simulink model "StabilityControlSystemMessy"  (R2023a)
settings: Solver=VariableStepAuto  StartTime=0.0  StopTime=10.0  RelTol=1e-3
libraries: simulink x2, slpidlib x1
settings Model: Creator=edill  LastModifiedBy=harshs
settings RTWCC: GPUComputeCapability=5.0
settings ConfigComp: CovBoundaryAbsTol=1.0e-5

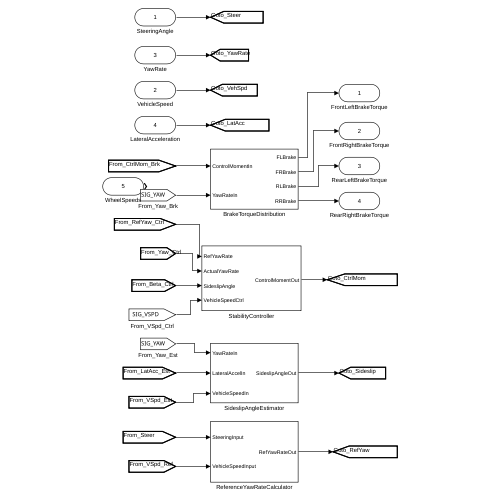
[thumbnail: Simulink's stored preview of the top-level diagram]
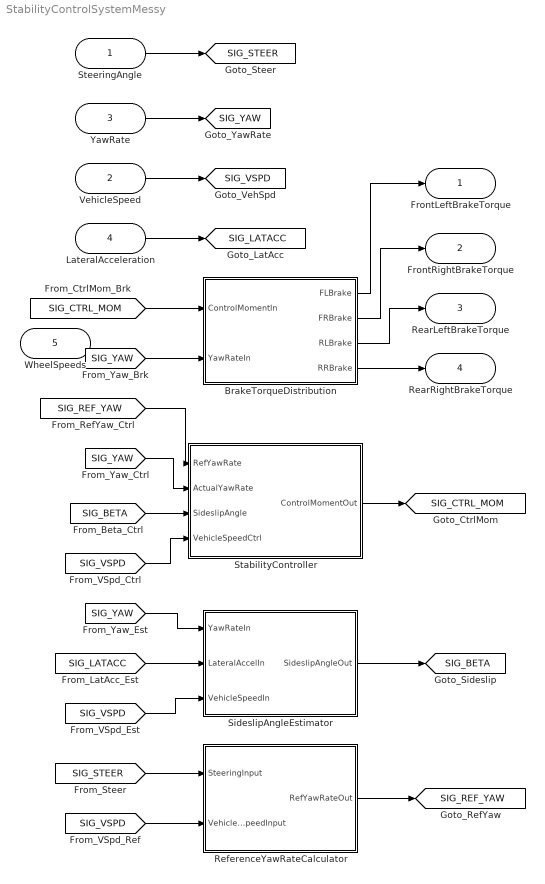
== system StabilityControlSystemMessy ==
  SteeringAngle : Inport
  VehicleSpeed : Inport  Port=2
  YawRate : Inport  Port=3
  LateralAcceleration : Inport  Port=4
  WheelSpeeds : Inport  Port=5  PortDimensions=4
  BrakeTorqueDistribution : Subsystem
  ReferenceYawRateCalculator : Subsystem
  SideslipAngleEstimator : Subsystem
  StabilityController : Subsystem
  FrontLeftBrakeTorque : Outport
  FrontRightBrakeTorque : Outport  Port=2
  RearLeftBrakeTorque : Outport  Port=3
  RearRightBrakeTorque : Outport  Port=4
  tag scope: SIG_BETA=global, SIG_CTRL_MOM=global, SIG_LATACC=global, SIG_REF_YAW=global, SIG_STEER=global, SIG_VSPD=global, SIG_YAW=global
  wires:
  [SIG_CTRL_MOM] -> BrakeTorqueDistribution/1(ControlMomentIn)
  VehicleSpeed/1 -> [SIG_VSPD]
  SteeringAngle/1 -> [SIG_STEER]
  ReferenceYawRateCalculator/1(RefYawRateOut) -> [SIG_REF_YAW]
  YawRate/1 -> [SIG_YAW]
  [SIG_YAW] -> StabilityController/2(ActualYawRate)
  LateralAcceleration/1 -> [SIG_LATACC]
  [SIG_YAW] -> BrakeTorqueDistribution/2(YawRateIn)
  [SIG_VSPD] -> SideslipAngleEstimator/3(VehicleSpeedIn)
  [SIG_REF_YAW] -> StabilityController/1(RefYawRate)
  [SIG_BETA] -> StabilityController/3(SideslipAngle)
  [SIG_VSPD] -> StabilityController/4(VehicleSpeedCtrl)
  [SIG_YAW] -> SideslipAngleEstimator/1(YawRateIn)
  [SIG_LATACC] -> SideslipAngleEstimator/2(LateralAccelIn)
  [SIG_STEER] -> ReferenceYawRateCalculator/1(SteeringInput)
  [SIG_VSPD] -> ReferenceYawRateCalculator/2(VehicleSpeedInput)
  BrakeTorqueDistribution/1(FLBrake) -> FrontLeftBrakeTorque/1
  BrakeTorqueDistribution/2(FRBrake) -> FrontRightBrakeTorque/1
  BrakeTorqueDistribution/3(RLBrake) -> RearLeftBrakeTorque/1
  BrakeTorqueDistribution/4(RRBrake) -> RearRightBrakeTorque/1
  StabilityController/1(ControlMomentOut) -> [SIG_CTRL_MOM]
  SideslipAngleEstimator/1(SideslipAngleOut) -> [SIG_BETA]

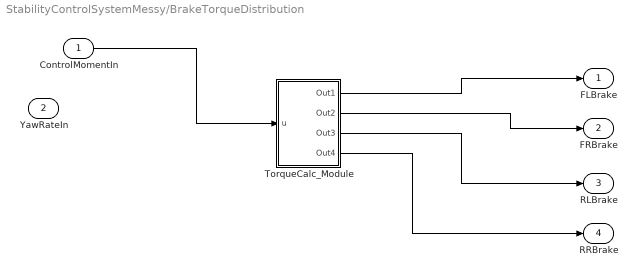
== system StabilityControlSystemMessy/BrakeTorqueDistribution ==
  ControlMomentIn : Inport
  YawRateIn : Inport  Port=2
  TorqueCalc_Module : Subsystem
  FLBrake : Outport
  FRBrake : Outport  Port=2
  RLBrake : Outport  Port=3
  RRBrake : Outport  Port=4
  wires:
  ControlMomentIn/1 -> TorqueCalc_Module/1(u)
  TorqueCalc_Module/1(Out1) -> FLBrake/1
  TorqueCalc_Module/2(Out2) -> FRBrake/1
  TorqueCalc_Module/3(Out3) -> RLBrake/1
  TorqueCalc_Module/4(Out4) -> RRBrake/1

== system StabilityControlSystemMessy/ReferenceYawRateCalculator ==
  SteeringInput : Inport
  VehicleSpeedInput : Inport  Port=2
  YawRateCalc_Core : Subsystem
  RefYawRateOut : Outport
  wires:
  SteeringInput/1 -> YawRateCalc_Core/1(In1)
  VehicleSpeedInput/1 -> YawRateCalc_Core/2(In2)
  YawRateCalc_Core/1(Out1) -> RefYawRateOut/1

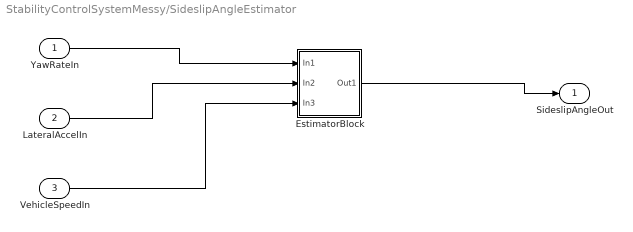
== system StabilityControlSystemMessy/SideslipAngleEstimator ==
  YawRateIn : Inport
  LateralAccelIn : Inport  Port=2
  VehicleSpeedIn : Inport  Port=3
  EstimatorBlock : Subsystem
  SideslipAngleOut : Outport
  wires:
  YawRateIn/1 -> EstimatorBlock/1(In1)
  LateralAccelIn/1 -> EstimatorBlock/2(In2)
  VehicleSpeedIn/1 -> EstimatorBlock/3(In3)
  EstimatorBlock/1(Out1) -> SideslipAngleOut/1

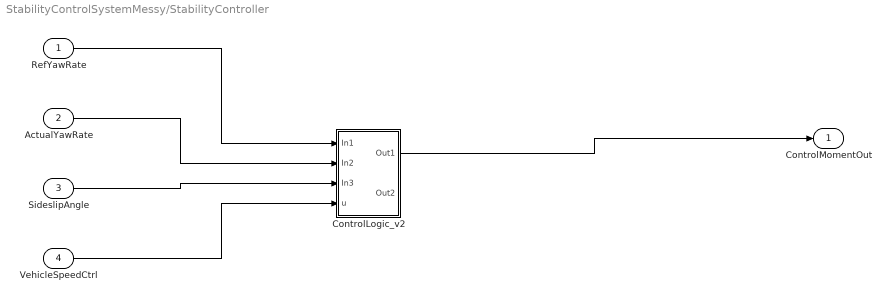
== system StabilityControlSystemMessy/StabilityController ==
  RefYawRate : Inport
  ActualYawRate : Inport  Port=2
  SideslipAngle : Inport  Port=3
  VehicleSpeedCtrl : Inport  Port=4
  ControlLogic_v2 : Subsystem
  ControlMomentOut : Outport
  wires:
  RefYawRate/1 -> ControlLogic_v2/1(In1)
  ActualYawRate/1 -> ControlLogic_v2/2(In2)
  SideslipAngle/1 -> ControlLogic_v2/3(In3)
  VehicleSpeedCtrl/1 -> ControlLogic_v2/4(u)
  ControlLogic_v2/1(Out1) -> ControlMomentOut/1

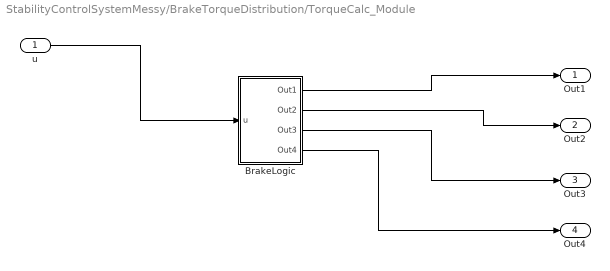
== system StabilityControlSystemMessy/BrakeTorqueDistribution/TorqueCalc_Module ==
  u : Inport
  BrakeLogic : Subsystem
  Out1 : Outport
  Out2 : Outport  Port=2
  Out3 : Outport  Port=3
  Out4 : Outport  Port=4
  wires:
  u/1 -> BrakeLogic/1(u)
  BrakeLogic/1(Out1) -> Out1/1
  BrakeLogic/2(Out2) -> Out2/1
  BrakeLogic/3(Out3) -> Out3/1
  BrakeLogic/4(Out4) -> Out4/1

== system StabilityControlSystemMessy/ReferenceYawRateCalculator/YawRateCalc_Core ==
  In1 : Inport
  In2 : Inport  Port=2
  MathOperations : Subsystem
  Out1 : Outport
  wires:
  In1/1 -> MathOperations/1(In1)
  In2/1 -> MathOperations/2(In2)
  MathOperations/1(Out1) -> Out1/1

== system StabilityControlSystemMessy/SideslipAngleEstimator/EstimatorBlock ==
  In1 : Inport
  In2 : Inport  Port=2
  In3 : Inport  Port=3
  IntegrationUnit : Subsystem
  Out1 : Outport
  wires:
  In1/1 -> IntegrationUnit/1(In1)
  In2/1 -> IntegrationUnit/2(In2)
  In3/1 -> IntegrationUnit/3(In3)
  IntegrationUnit/1(Out1) -> Out1/1

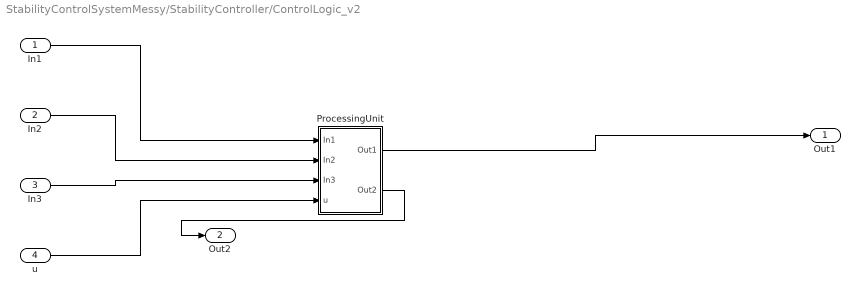
== system StabilityControlSystemMessy/StabilityController/ControlLogic_v2 ==
  In1 : Inport
  In2 : Inport  Port=2
  In3 : Inport  Port=3
  u : Inport  Port=4
  ProcessingUnit : Subsystem
  Out1 : Outport
  Out2 : Outport  Port=2
  wires:
  In1/1 -> ProcessingUnit/1(In1)
  In2/1 -> ProcessingUnit/2(In2)
  In3/1 -> ProcessingUnit/3(In3)
  u/1 -> ProcessingUnit/4(u)
  ProcessingUnit/1(Out1) -> Out1/1
  ProcessingUnit/2(Out2) -> Out2/1

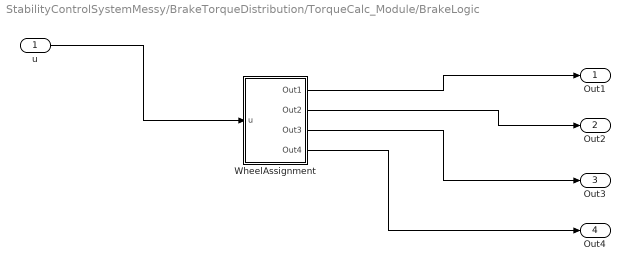
== system StabilityControlSystemMessy/BrakeTorqueDistribution/TorqueCalc_Module/BrakeLogic ==
  u : Inport
  WheelAssignment : Subsystem
  Out1 : Outport
  Out2 : Outport  Port=2
  Out3 : Outport  Port=3
  Out4 : Outport  Port=4
  wires:
  u/1 -> WheelAssignment/1(u)
  WheelAssignment/1(Out1) -> Out1/1
  WheelAssignment/2(Out2) -> Out2/1
  WheelAssignment/3(Out3) -> Out3/1
  WheelAssignment/4(Out4) -> Out4/1

== system StabilityControlSystemMessy/ReferenceYawRateCalculator/YawRateCalc_Core/MathOperations ==
  In1 : Inport
  In2 : Inport  Port=2
  CalcEngine : Subsystem
  Out1 : Outport
  wires:
  In1/1 -> CalcEngine/1(In1)
  In2/1 -> CalcEngine/2(In2)
  CalcEngine/1(Out1) -> Out1/1

== system StabilityControlSystemMessy/SideslipAngleEstimator/EstimatorBlock/IntegrationUnit ==
  In1 : Inport
  In2 : Inport  Port=2
  In3 : Inport  Port=3
  SignalProcessing : Subsystem
  Out1 : Outport
  wires:
  In1/1 -> SignalProcessing/1(In1)
  In2/1 -> SignalProcessing/2(In2)
  In3/1 -> SignalProcessing/3(In3)
  SignalProcessing/1(Out1) -> Out1/1

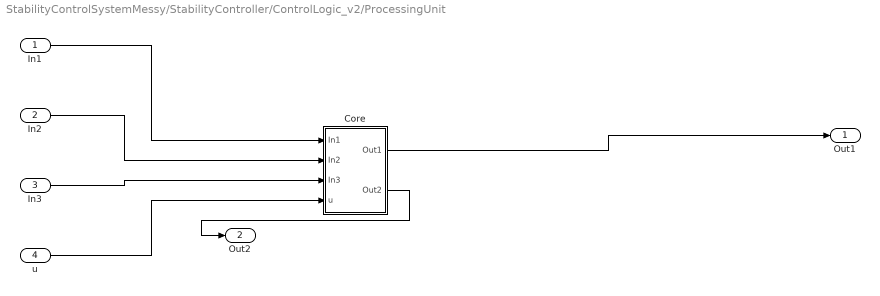
== system StabilityControlSystemMessy/StabilityController/ControlLogic_v2/ProcessingUnit ==
  In1 : Inport
  In2 : Inport  Port=2
  In3 : Inport  Port=3
  u : Inport  Port=4
  Core : Subsystem
  Out1 : Outport
  Out2 : Outport  Port=2
  wires:
  In1/1 -> Core/1(In1)
  In2/1 -> Core/2(In2)
  In3/1 -> Core/3(In3)
  u/1 -> Core/4(u)
  Core/1(Out1) -> Out1/1
  Core/2(Out2) -> Out2/1

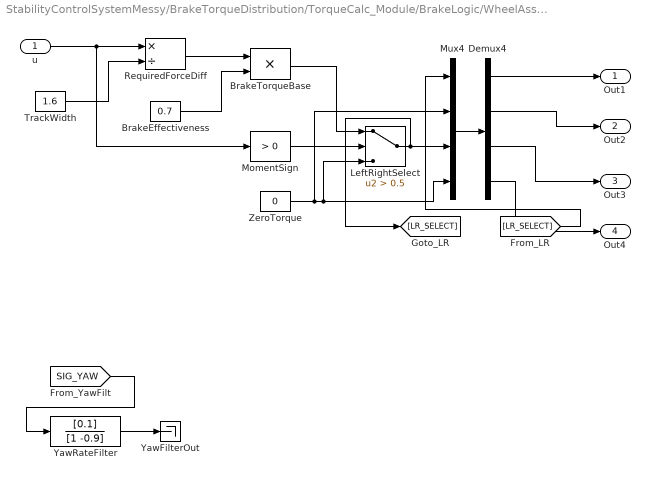
== system StabilityControlSystemMessy/BrakeTorqueDistribution/TorqueCalc_Module/BrakeLogic/WheelAssignment ==
  u : Inport
  BrakeEffectiveness : Constant  Value=0.7
  BrakeTorqueBase : Product
  Demux4 : Demux
  LeftRightSelect : Switch  Criteria=u2 > Threshold  Threshold=0.5  SaturateOnIntegerOverflow=off  InputSameDT=off
  MomentSign : simulink/Logic and Bit Operations/Compare To Zero  relop=>  OutDataTypeStr=boolean
  Mux4 : Mux
  RequiredForceDiff : Product  Inputs=*/
  TrackWidth : Constant  Value=1.6
  YawFilterOut : Terminator
  YawRateFilter : DiscreteFilter  Numerator=[0.1]  Denominator=[1 -0.9]
  ZeroTorque : Constant  Value=0
  Out1 : Outport
  Out2 : Outport  Port=2
  Out3 : Outport  Port=3
  Out4 : Outport  Port=4
  wires:
  MomentSign/1 -> LeftRightSelect/2
  u/1 -> MomentSign/1, RequiredForceDiff/1
  LeftRightSelect/1 -> Mux4/3, [LR_SELECT]
  ZeroTorque/1 -> Mux4/4, LeftRightSelect/3, Mux4/2
  Mux4/1 -> Demux4/1
  BrakeTorqueBase/1 -> LeftRightSelect/1
  TrackWidth/1 -> RequiredForceDiff/2
  RequiredForceDiff/1 -> BrakeTorqueBase/1
  BrakeEffectiveness/1 -> BrakeTorqueBase/2
  Demux4/1 -> Out1/1
  Demux4/3 -> Out3/1
  Demux4/4 -> Out4/1
  Demux4/2 -> Out2/1
  [LR_SELECT] -> Mux4/1
  [SIG_YAW] -> YawRateFilter/1
  YawRateFilter/1 -> YawFilterOut/1

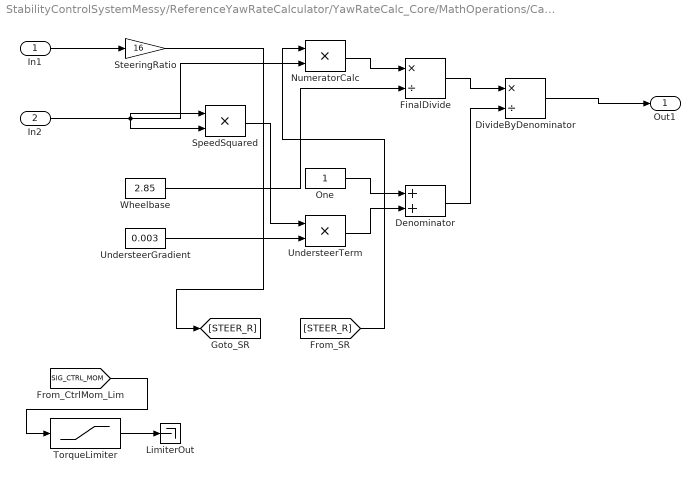
== system StabilityControlSystemMessy/ReferenceYawRateCalculator/YawRateCalc_Core/MathOperations/CalcEngine ==
  In1 : Inport
  In2 : Inport  Port=2
  Denominator : Sum
  DivideByDenominator : Product  Inputs=*/
  FinalDivide : Product  Inputs=*/
  LimiterOut : Terminator
  NumeratorCalc : Product
  One : Constant
  SpeedSquared : Product
  SteeringRatio : Gain  Gain=16
  TorqueLimiter : Saturate  UpperLimit=5000  LowerLimit=-5000
  UndersteerGradient : Constant  Value=0.003
  UndersteerTerm : Product
  Wheelbase : Constant  Value=2.85
  Out1 : Outport
  wires:
  One/1 -> Denominator/1
  UndersteerTerm/1 -> Denominator/2
  SpeedSquared/1 -> UndersteerTerm/1
  UndersteerGradient/1 -> UndersteerTerm/2
  FinalDivide/1 -> DivideByDenominator/1
  In2/1 -> NumeratorCalc/2, SpeedSquared/1, SpeedSquared/2
  NumeratorCalc/1 -> FinalDivide/1
  Wheelbase/1 -> FinalDivide/2
  Denominator/1 -> DivideByDenominator/2
  DivideByDenominator/1 -> Out1/1
  In1/1 -> SteeringRatio/1
  SteeringRatio/1 -> [STEER_R]
  [STEER_R] -> NumeratorCalc/1
  [SIG_CTRL_MOM] -> TorqueLimiter/1
  TorqueLimiter/1 -> LimiterOut/1

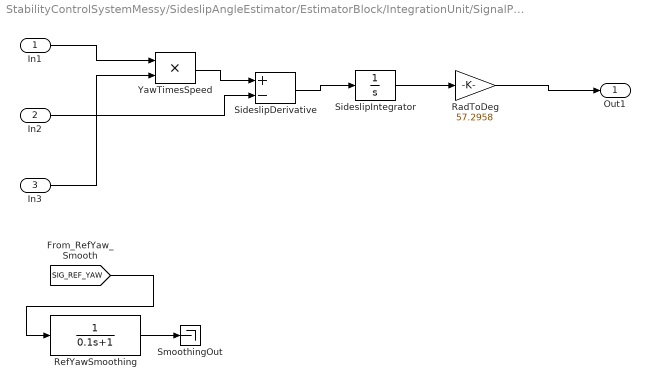
== system StabilityControlSystemMessy/SideslipAngleEstimator/EstimatorBlock/IntegrationUnit/SignalProcessing ==
  In1 : Inport
  In2 : Inport  Port=2
  In3 : Inport  Port=3
  RadToDeg : Gain  Gain=57.2958
  RefYawSmoothing : TransferFcn  Denominator=[0.1 1]
  SideslipDerivative : Sum  Inputs=+-
  SideslipIntegrator : Integrator
  SmoothingOut : Terminator
  YawTimesSpeed : Product
  Out1 : Outport
  wires:
  SideslipDerivative/1 -> SideslipIntegrator/1
  SideslipIntegrator/1 -> RadToDeg/1
  YawTimesSpeed/1 -> SideslipDerivative/1
  In3/1 -> YawTimesSpeed/2
  RadToDeg/1 -> Out1/1
  In2/1 -> SideslipDerivative/2
  In1/1 -> YawTimesSpeed/1
  [SIG_REF_YAW] -> RefYawSmoothing/1
  RefYawSmoothing/1 -> SmoothingOut/1

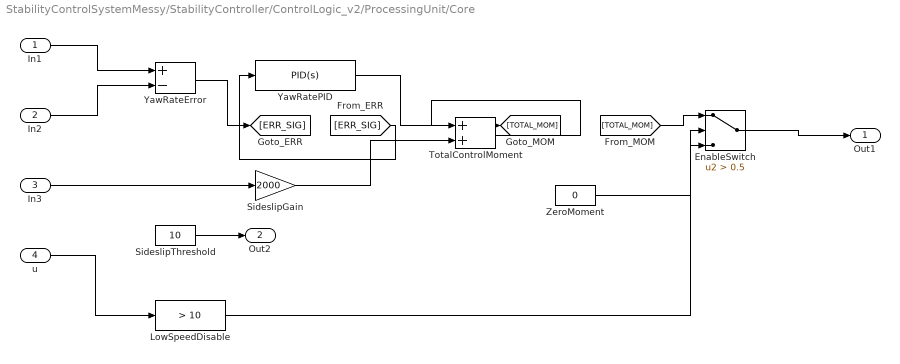
== system StabilityControlSystemMessy/StabilityController/ControlLogic_v2/ProcessingUnit/Core ==
  In1 : Inport
  In2 : Inport  Port=2
  In3 : Inport  Port=3
  u : Inport  Port=4
  EnableSwitch : Switch  Criteria=u2 > Threshold  Threshold=0.5  SaturateOnIntegerOverflow=off  InputSameDT=off
  LowSpeedDisable : simulink/Logic and Bit Operations/Compare To Constant  relop=>  const=10  OutDataTypeStr=boolean
  SideslipGain : Gain  Gain=2000
  SideslipThreshold : Constant  Value=10
  TotalControlMoment : Sum
  YawRateError : Sum  Inputs=+-
  YawRatePID : slpidlib/PID Controller  Controller=PID  Form=Parallel  TimeDomain=Continuous-time  UseExternalTs=off  SampleTime=-1  IntegratorMethod=Forward Euler  FilterMethod=Forward Euler  ControllerParametersSource=internal  P=5000  I=1000  UseKiTs=off  D=100  N=100  UseFilter=on  TunerSelectOption=Transfer Function Based (PID Tuner App)  InitialConditionSource=internal  InitialConditionForIntegrator=0  InitialConditionForFilter=0  DifferentiatorICPrevScaledInput=0  ExternalReset=none  TrackingMode=off  Kt=1  LimitOutput=off  SatLimitsSource=internal  UpperSaturationLimit=inf  LowerSaturationLimit=-inf  LinearizeAsGain=on  AntiWindupMode=none  Kb=1  LimitIntegrator=off  UpperIntegratorSaturationLimit=inf  LowerIntegratorSaturationLimit=-inf  POutMin=[]  POutMax=[]  IOutMin=[]  IOutMax=[]  DOutMin=[]  DOutMax=[]  NOutMin=[]  NOutMax=[]  SumOutMin=[]  SumOutMax=[]  SaturationOutMin=[]  SaturationOutMax=[]  PParamMin=[]  PParamMax=[]  IParamMin=[]  IParamMax=[]  DParamMin=[]  DParamMax=[]  NParamMin=[]  NParamMax=[]  KbParamMin=[]  KbParamMax=[]  KtParamMin=[]  KtParamMax=[]  KbOutMin=[]  KbOutMax=[]  KtOutMin=[]  KtOutMax=[]  IntegratorOutMin=[]  IntegratorOutMax=[]  FilterOutMin=[]  FilterOutMax=[]  SumI1OutMin=[]  SumI1OutMax=[]  SumI2OutMin=[]  SumI2OutMax=[]  SumI3OutMin=[]  SumI3OutMax=[]  SumI4OutMin=[]  SumI4OutMax=[]  SumDOutMin=[]  SumDOutMax=[]  DifferentiatorOutMin=[]  DifferentiatorOutMax=[]  FilterDiffOutCoefMin=[]  FilterDiffOutCoefMax=[]  ReciprocalOutMin=[]  ReciprocalOutMax=[]  SumDenOutMin=[]  SumDenOutMax=[]  SumNumOutMin=[]  SumNumOutMax=[]  DivideOutMin=[]  DivideOutMax=[]  UdiffTsProdOutMin=[]  UdiffTsProdOutMax=[]  NTsProdOutMin=[]  NTsProdOutMax=[]  UintegralTsProdOutMin=[]  UintegralTsProdOutMax=[]  UngainTsProdOutMin=[]  UngainTsProdOutMax=[]  ClampingZeroOutDataTypeStr=Inherit: Inherit via back propagation  ClampingZeroOutMin=[]  ClampingZeroOutMax=[]  FilterDenConstantOutDataTypeStr=Inherit: Inherit via back propagation  FilterDenConstantOutMin=[]  FilterDenConstantOutMax=[]  PCopyOutDataTypeStr=Inherit: Inherit via back propagation  PCopyOutMin=[]  PCopyOutMax=[]  NCopyOutDataTypeStr=Inherit: Inherit via back propagation  NCopyOutMin=[]  NCopyOutMax=[]  IntegratorContinuousStateAttributes=''  IntegratorStateMustResolveToSignalObject=off  IntegratorRTWStateStorageClass=Auto  FilterContinuousStateAttributes=''  FilterStateMustResolveToSignalObject=off  FilterRTWStateStorageClass=Auto  ParallelPVariant=InternalParameters  IdealPVariant=Disabled  IVariant=InternalParameters  DVariant=InternalParameters  IntegratorVariant=Continuous  SatVariant=Disabled  AWVariant=Passthrough  PCopyVariant=Disabled  TRVariant=Disabled  FdbkBlocksVariant=Forward  IdealPFdbkVariant=Disabled  SatFdbkVariant=Disabled  DerivativeFilterVariant=ContFilter  NVariant=InternalParameters  NCopyVariant=Disabled  FilterICVariant=InternalICsFilter  IntegratorICVariant=InternalICs  ExternalResetVariant=Disabled  TRSumVariant=Passthrough  SumFdbkVariant=Disabled  SumVariant=Sum_PID  TsampFilterVariant=InternalTs  TsampNgainVariant=Passthrough  TsampIntegralVariant=Disabled_SignalSpec  ExternalSaturationOutDataTypeStr=Inherit: Same as second input
  ZeroMoment : Constant  Value=0
  Out1 : Outport
  Out2 : Outport  Port=2
  wires:
  LowSpeedDisable/1 -> EnableSwitch/2
  SideslipGain/1 -> TotalControlMoment/2
  u/1 -> LowSpeedDisable/1
  ZeroMoment/1 -> EnableSwitch/3
  SideslipThreshold/1 -> Out2/1
  YawRatePID/1 -> TotalControlMoment/1
  In1/1 -> YawRateError/1
  EnableSwitch/1 -> Out1/1
  In3/1 -> SideslipGain/1
  In2/1 -> YawRateError/2
  YawRateError/1 -> [ERR_SIG]
  [ERR_SIG] -> YawRatePID/1
  TotalControlMoment/1 -> [TOTAL_MOM]
  [TOTAL_MOM] -> EnableSwitch/1
